simulink library "led_attivita"  (R2024b)
settings: Solver=VariableStepAuto  StartTime=0.0  StopTime=10.0  RelTol=1e-3
settings Model: Creator=mainuser  LastModifiedBy=mainuser

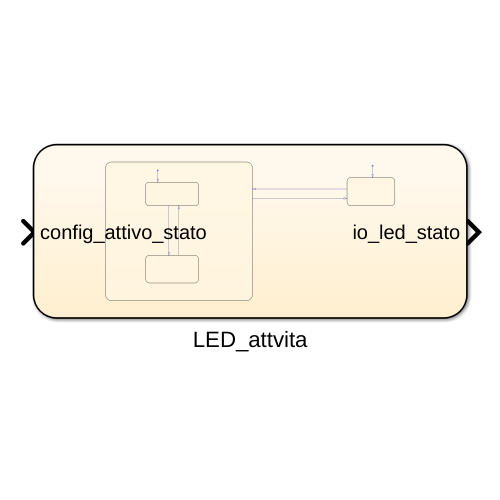
[thumbnail: Simulink's stored preview of the top-level diagram]
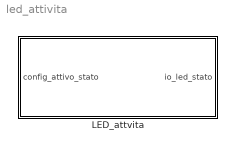
== system led_attivita ==
  LED_attvita : Stateflow chart  TreatAsAtomicUnit=on

== stateflow chart led_attivita/LED_attvita ==
  state Attivo
    state Attivo_ON
      en: io_led_stato=1
    state Attivo_OFF
      en: io_led_stato=0
    (default) -> Attivo_ON
    Attivo_ON -> Attivo_OFF : after(0.5,sec)
    Attivo_OFF -> Attivo_ON : after(0.5,sec)
  state Inattivo
    en: io_led_stato=0
  (default) -> Inattivo
  Inattivo -> Attivo : [config_attivo_stato==true]
  Attivo -> Inattivo : [config_attivo_stato==false]
  data: io_led_stato output; config_attivo_stato input
